simulink model "Modelling_DC_Motor"  (R2016a)
settings: Solver=ode23tb  StartTime=0.0  StopTime=10  RelTol=1e-3
undefined symbols (not defined in the file or in its folder): B, J, K, L, R
libraries: simulink x1
settings Model: Creator=faiq1  LastModifiedBy=faiq1

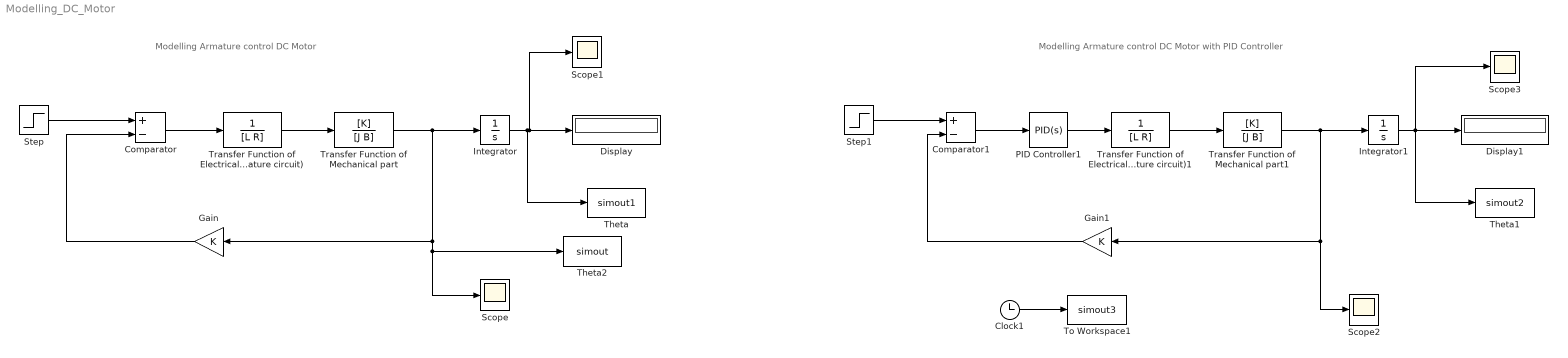
== system Modelling_DC_Motor ==
  note: Modelling Armature control DC Motor
  note: Modelling Armature control DC Motor
      | with PID Controller
  Clock1 : Clock
  Comparator : Sum  Inputs=+-
  Comparator1 : Sum  Inputs=+-
  Display : Display
  Display1 : Display
  Gain : Gain  Gain=K
  Gain1 : Gain  Gain=K
  Integrator : Integrator
  Integrator1 : Integrator
  PID Controller1 : simulink/Continuous/PID Controller  Controller=PID  TimeDomain=Continuous-time  SampleTime=-1  IntegratorMethod=Forward Euler  FilterMethod=Forward Euler  Form=Parallel  UseFilter=on  ControllerParametersSource=internal  P=1821.23311115773  I=5127.18575823411  D=95.7750934355267  N=37.1993217775763  InitialConditionSource=internal  InitialConditionForIntegrator=0  InitialConditionForFilter=0  ExternalReset=none  LimitOutput=off  UpperSaturationLimit=inf  LowerSaturationLimit=-inf  LinearizeAsGain=on  AntiWindupMode=none  Kb=1  TrackingMode=off  Kt=1  PParamMin=[]  PParamMax=[]  IParamMin=[]  IParamMax=[]  DParamMin=[]  DParamMax=[]  NParamMin=[]  NParamMax=[]  KbParamMin=[]  KbParamMax=[]  KtParamMin=[]  KtParamMax=[]  POutMin=[]  POutMax=[]  IOutMin=[]  IOutMax=[]  DOutMin=[]  DOutMax=[]  NOutMin=[]  NOutMax=[]  KbOutMin=[]  KbOutMax=[]  KtOutMin=[]  KtOutMax=[]  IntegratorOutMin=[]  IntegratorOutMax=[]  FilterOutMin=[]  FilterOutMax=[]  SumOutMin=[]  SumOutMax=[]  SumI1OutMin=[]  SumI1OutMax=[]  SumI2OutMin=[]  SumI2OutMax=[]  SumI3OutMin=[]  SumI3OutMax=[]  SumDOutMin=[]  SumDOutMax=[]  SaturationOutMin=[]  SaturationOutMax=[]  IntegratorContinuousStateAttributes=''  IntegratorStateMustResolveToSignalObject=off  IntegratorRTWStateStorageClass=Auto  FilterContinuousStateAttributes=''  FilterStateMustResolveToSignalObject=off  FilterRTWStateStorageClass=Auto  DifferentiatorICPrevScaledInput=0  DifferentiatorOutMin=[]  DifferentiatorOutMax=[]
  Scope{,1..3} (4 alike) : Scope
  Step : Step  After=10  SampleTime=0
  Step1 : Step  After=200  SampleTime=0
  Theta : ToWorkspace  VariableName=simout1  SaveFormat=Timeseries  SampleTime=-1
  Theta1 : ToWorkspace  VariableName=simout2  SaveFormat=Timeseries  SampleTime=-1
  Theta2 : ToWorkspace  VariableName=simout  SaveFormat=Timeseries  SampleTime=-1
  To Workspace1 : ToWorkspace  VariableName=simout3  SaveFormat=Timeseries  SampleTime=-1
  Transfer Function of Electrical part (Armature circuit) : TransferFcn  Denominator=[L R]
  Transfer Function of Electrical part (Armature circuit)1 : TransferFcn  Denominator=[L R]
  Transfer Function of Mechanical part : TransferFcn  Numerator=[K]  Denominator=[J B]
  Transfer Function of Mechanical part1 : TransferFcn  Numerator=[K]  Denominator=[J B]
  wires:
  Step/1 -> Comparator/1
  Gain/1 -> Comparator/2
  Comparator/1 -> Transfer Function of Electrical part (Armature circuit)/1
  Transfer Function of Electrical part (Armature circuit)/1 -> Transfer Function of Mechanical part/1
  Transfer Function of Mechanical part/1 -> Integrator/1, Theta2/1, Scope/1, Gain/1
  Integrator/1 -> Scope1/1, Display/1, Theta/1
  Step1/1 -> Comparator1/1
  Gain1/1 -> Comparator1/2
  Comparator1/1 -> PID Controller1/1
  Transfer Function of Electrical part (Armature circuit)1/1 -> Transfer Function of Mechanical part1/1
  Transfer Function of Mechanical part1/1 -> Integrator1/1, Scope2/1, Gain1/1
  Integrator1/1 -> Scope3/1, Display1/1, Theta1/1
  Clock1/1 -> To Workspace1/1
  PID Controller1/1 -> Transfer Function of Electrical part (Armature circuit)1/1
